simulink model "sldemo_foreach_repeat_tile"  (Simulink 7.6)
settings: Solver=FixedStepDiscrete  StartTime=0.0  StopTime=1.0  FixedStep=0.2  RelTol=1e-3
settings Model: Creator=The MathWorks Inc.
settings DataIOCC: SaveFormat=Structure
settings OptimizationCC: OptimizeModelRefInitCode=on  LifeSpan=1
settings RTWCC: SystemTargetFile=ert.tlc  TemplateMakefile=ert_default_tmf  Description=Real-Time Workshop Embedded Coder  GenerateReport=on  ProcessScript=ert_make_rtw_hook  IncludeHyperlinkInReport=on  LaunchReport=on
settings CodeAppCC: IgnoreCustomStorageClasses=off
settings ERTTargetCC: MultiwordLength=2048  GenerateSampleERTMain=on  MatFileLogging=on  SupportVariableSizeSignals=on  ERTCustomFileTemplate=example_file_process.tlc  ConvertIfToSwitch=off

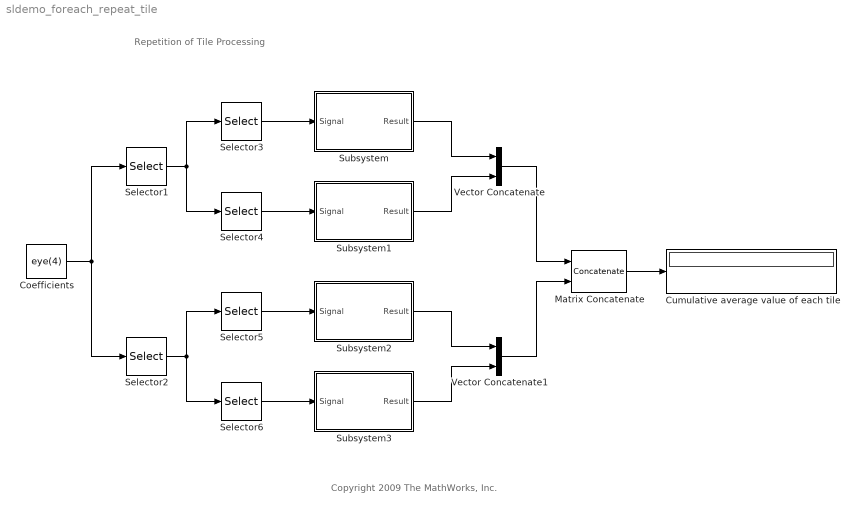
== system sldemo_foreach_repeat_tile ==
  note: Repetition of Tile Processing
  note: Copyright 2009 The MathWorks, Inc.
  Coefficients : Constant  Value=eye(4)
  Cumulative average value of each tile : Display
  Matrix Concatenate : Concatenate  Mode=Multidimensional array  ConcatenateDimension=2
  Selector1 : Selector  NumberOfDimensions=2  InputPortWidth=3  IndexOptions=Index vector (dialog),Select all  Indices=[1 2],1  OutputSizes=1,1
  Selector2 : Selector  NumberOfDimensions=2  InputPortWidth=3  IndexOptions=Index vector (dialog),Select all  Indices=[3 4],1  OutputSizes=1,1
  Selector3 : Selector  NumberOfDimensions=2  InputPortWidth=3  IndexOptions=Select all,Index vector (dialog)  Indices=[1 2],[1 2]  OutputSizes=1,1
  Selector4 : Selector  NumberOfDimensions=2  InputPortWidth=3  IndexOptions=Select all,Index vector (dialog)  Indices=[1 2],[3 4]  OutputSizes=1,1
  Selector5 : Selector  NumberOfDimensions=2  InputPortWidth=3  IndexOptions=Select all,Index vector (dialog)  Indices=[1 2],[1 2]  OutputSizes=1,1
  Selector6 : Selector  NumberOfDimensions=2  InputPortWidth=3  IndexOptions=Select all,Index vector (dialog)  Indices=[1 2],[3 4]  OutputSizes=1,1
  Subsystem : Subsystem
  Subsystem1 : Subsystem
  Subsystem2 : Subsystem
  Subsystem3 : Subsystem
  Vector Concatenate : Concatenate  Mode=Vector
  Vector Concatenate1 : Concatenate  Mode=Vector
  wires:
  Coefficients/1 -> Selector1/1, Selector2/1
  Selector1/1 -> Selector3/1, Selector4/1
  Selector2/1 -> Selector5/1, Selector6/1
  Selector3/1 -> Subsystem/1(Signal)
  Subsystem2/1(Result) -> Vector Concatenate1/1
  Subsystem3/1(Result) -> Vector Concatenate1/2
  Selector5/1 -> Subsystem2/1(Signal)
  Selector6/1 -> Subsystem3/1(Signal)
  Selector4/1 -> Subsystem1/1(Signal)
  Subsystem/1(Result) -> Vector Concatenate/1
  Subsystem1/1(Result) -> Vector Concatenate/2
  Vector Concatenate1/1 -> Matrix Concatenate/2
  Vector Concatenate/1 -> Matrix Concatenate/1
  Matrix Concatenate/1 -> Cumulative average value of each tile/1

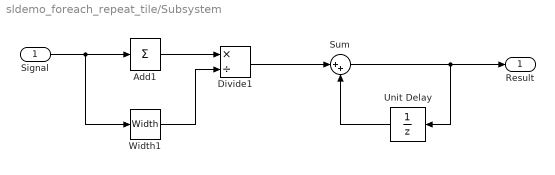
== system sldemo_foreach_repeat_tile/Subsystem ==
  Signal : Inport
  Add1 : Sum  Inputs=+
  Divide1 : Product  Inputs=*/
  Sum : Sum  Inputs=|++
  Unit Delay : UnitDelay  SampleTime=-1
  Width1 : Width
  Result : Outport
  wires:
  Signal/1 -> Add1/1, Width1/1
  Add1/1 -> Divide1/1
  Width1/1 -> Divide1/2
  Divide1/1 -> Sum/1
  Sum/1 -> Result/1, Unit Delay/1
  Unit Delay/1 -> Sum/2

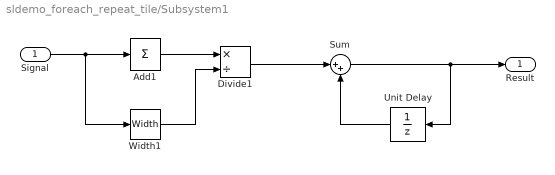
== system sldemo_foreach_repeat_tile/Subsystem1 ==
  Signal : Inport
  Add1 : Sum  Inputs=+
  Divide1 : Product  Inputs=*/
  Sum : Sum  Inputs=|++
  Unit Delay : UnitDelay  SampleTime=-1
  Width1 : Width
  Result : Outport
  wires:
  Unit Delay/1 -> Sum/2
  Sum/1 -> Unit Delay/1, Result/1
  Divide1/1 -> Sum/1
  Width1/1 -> Divide1/2
  Add1/1 -> Divide1/1
  Signal/1 -> Width1/1, Add1/1

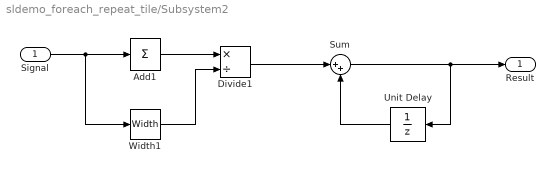
== system sldemo_foreach_repeat_tile/Subsystem2 ==
  Signal : Inport
  Add1 : Sum  Inputs=+
  Divide1 : Product  Inputs=*/
  Sum : Sum  Inputs=|++
  Unit Delay : UnitDelay  SampleTime=-1
  Width1 : Width
  Result : Outport
  wires:
  Signal/1 -> Add1/1, Width1/1
  Add1/1 -> Divide1/1
  Width1/1 -> Divide1/2
  Divide1/1 -> Sum/1
  Sum/1 -> Result/1, Unit Delay/1
  Unit Delay/1 -> Sum/2

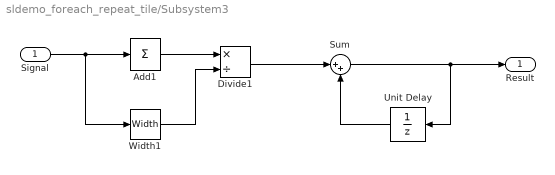
== system sldemo_foreach_repeat_tile/Subsystem3 ==
  Signal : Inport
  Add1 : Sum  Inputs=+
  Divide1 : Product  Inputs=*/
  Sum : Sum  Inputs=|++
  Unit Delay : UnitDelay  SampleTime=-1
  Width1 : Width
  Result : Outport
  wires:
  Unit Delay/1 -> Sum/2
  Sum/1 -> Unit Delay/1, Result/1
  Divide1/1 -> Sum/1
  Width1/1 -> Divide1/2
  Add1/1 -> Divide1/1
  Signal/1 -> Width1/1, Add1/1
